simulink model "sampleModel2199"  (R2022a)
settings: Solver=FixedStepAuto  StartTime=0.0  StopTime=10.0  RelTol=1e-3
undefined symbols (not defined in the file): DiscIntNeverNeededParam, Newton, Raphson
libraries: simulink x64, slpidlib x16
(part 1 of 3)
settings Model: SimulationMode=software-in-the-loop (sil)  Creator=lenovo  LastModifiedBy=TSMC
settings DataIOCC: InspectSignalLogs=on  SignalLoggingName=logsOut
settings OptimizationCC: DefaultParameterBehavior=Inlined  EnhancedBackFolding=on  PassReuseOutputArgsAs=Individual arguments  ZeroExternalMemoryAtStartup=off  ZeroInternalMemoryAtStartup=off  OptimizeBlockOrder=speed  DifferentSizesBufferReuse=on  OptimizationCustomize=off  EfficientTunableParamExpr=on
settings DebuggingCC: ParameterTunabilityLossMsg=error  UnconnectedInputMsg=warning  UnconnectedOutputMsg=warning  UnconnectedLineMsg=warning
settings ModelReferenceCC: UpdateModelReferenceTargets=Force
settings SFSimCC: MATLABDynamicMemAlloc=off
settings RTWCC: SystemTargetFile=ert.tlc  TemplateMakefile=ert_default_tmf  GenerateReport=on  IncludeHyperlinkInReport=on  GenerateTraceInfo=on  DLArmComputeVersion=19.05
settings CodeAppCC: ForceParamTrailComments=on  IgnoreCustomStorageClasses=off  OperatorAnnotations=on  SimulinkDataObjDesc=on  SFDataObjDesc=on  InsertBlockDesc=on
settings ERTTargetCC: TargetLangStandard=C99 (ISO)  GenerateSampleERTMain=on  SupportContinuousTime=on  InlinedParameterPlacement=NonHierarchical  ERTCustomFileTemplate=example_file_process.tlc

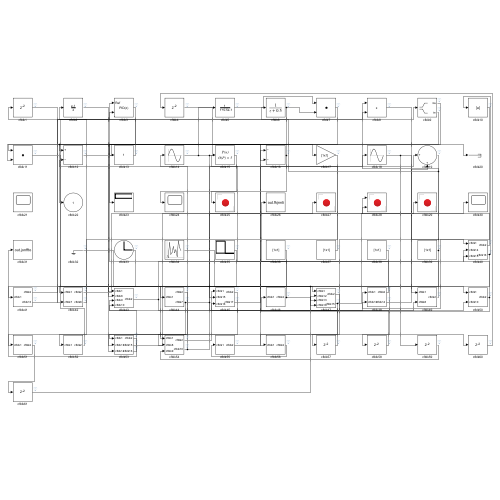
[thumbnail: Simulink's stored preview of the top-level diagram]
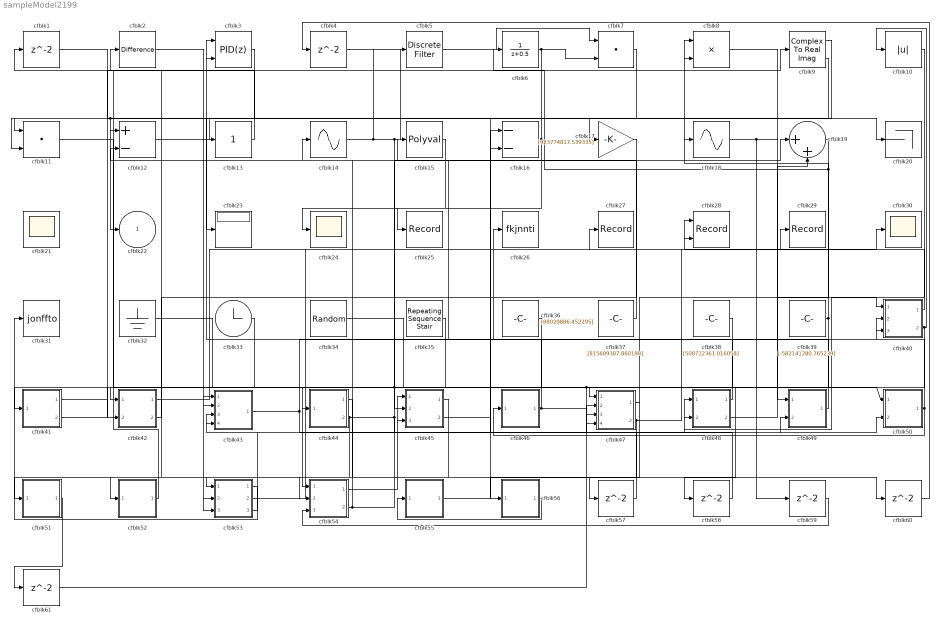
== system sampleModel2199 ==
  cfblk{1,4,57..61} (7 alike) : Delay  SampleTime=1
  cfblk10 : Abs  SaturateOnIntegerOverflow=off
  cfblk11 : DotProduct  OutDataTypeStr=Inherit: Inherit via internal rule
  cfblk12 : Sum  Inputs=+-
  cfblk13 : simulink/Math Operations/Slider Gain  gain=1  low=0  high=2
  cfblk14 : Sin  TimeSource=Use external signal  SampleTime=0
  cfblk15 : Polyval  Coefs=[ +2.081618890e-019, -1.441693666e-014, +4.719686976e-010, -8.536869453e-006, +1.621573104e-001, -8.087801117e+001 ]
  cfblk16 : Sum  Inputs=--
  cfblk17 : Gain  Gain=[923774817.539335]
  cfblk18 : Sin  TimeSource=Use external signal  SampleTime=0
  cfblk19 : Sum  Inputs=|++
  cfblk2 : simulink/Discrete/Difference  ICPrevInput=0.0  OutMin=[]  OutMax=[]  OutDataTypeStr=Inherit: Inherit via back propagation  OutDataType=fixdt(1, 16)  OutScaling=2^-10  DoSatur=off
  cfblk20 : Terminator
  cfblk21 : Scope
      settings: Floating=on
  cfblk23 : Display
  cfblk24 : Scope
  cfblk25 : Record  FileSettingsInternal="{\"entries\":[{\"content\":{\"excelSettings\":{\"content\":{},\"type\":\"Streamout.ExcelSettings\"}},\"type\":\"Streamout.FileSettingStorage\",\"uuid\":\"e2bdf832-fa04-45a0-9737-202340bf4c1e\"}],\"packageUris\":[\"http://schema.mathworks.com/mf0/streamout_blocks/R2020a\"],\"version\":\"1.0\"}"  SignalsInternal="{\"entries\":[{\"content\":{\"signals\":[]},\"type\":\"RecordBlkView.InputSignals\",\"uuid\":\"caab4e54-0413-4384-8605-d26ba1fc89d5\"}],\"packageUris\":[\"http://schema.mathworks.com/mf0/streamout_blocks/R2020a\"],\"version\":\"1.0\"}"  VisualizationBindings="{\"sparklinesplugin\":{\"info\":[{\"bindingParametersList\":[],\"subplotID\":1}]}}"
  cfblk26 : ToWorkspace  VariableName=fkjnnti  SaveFormat=Timeseries  SampleTime=-1
  cfblk27 : Record  FileSettingsInternal="{\"entries\":[{\"content\":{\"excelSettings\":{\"content\":{},\"type\":\"Streamout.ExcelSettings\"}},\"type\":\"Streamout.FileSettingStorage\",\"uuid\":\"b3a37654-cf2f-4752-9820-15f634001c55\"}],\"packageUris\":[\"http://schema.mathworks.com/mf0/streamout_blocks/R2020a\"],\"version\":\"1.0\"}"  SignalsInternal="{\"entries\":[{\"content\":{\"signals\":[]},\"type\":\"RecordBlkView.InputSignals\",\"uuid\":\"67388c61-a990-4278-b841-d462b1e08af4\"}],\"packageUris\":[\"http://schema.mathworks.com/mf0/streamout_blocks/R2020a\"],\"version\":\"1.0\"}"  VisualizationBindings="{\"sparklinesplugin\":{\"info\":[{\"bindingParametersList\":[],\"subplotID\":1}]}}"
  cfblk28 : Record  FileSettingsInternal="{\"entries\":[{\"content\":{\"excelSettings\":{\"content\":{},\"type\":\"Streamout.ExcelSettings\"}},\"type\":\"Streamout.FileSettingStorage\",\"uuid\":\"9d0e44ae-21f0-49fd-83ab-d770f6f5ba27\"}],\"packageUris\":[\"http://schema.mathworks.com/mf0/streamout_blocks/R2020a\"],\"version\":\"1.0\"}"  Layout=[1 1]  SignalsInternal="{\"entries\":[{\"content\":{\"signals\":[]},\"type\":\"RecordBlkView.InputSignals\",\"uuid\":\"6b70960c-b6c1-44c9-85c3-124069d1ad3e\"}],\"packageUris\":[\"http://schema.mathworks.com/mf0/streamout_blocks/R2020a\"],\"version\":\"1.0\"}"  VisualizationBindings="{\"xyplotplugin\":{\"info\":[{\"series\":[],\"subplotID\":1}]}}"  CompatibilityTag=XY  st=-1
  cfblk29 : Record  FileSettingsInternal="{\"entries\":[{\"content\":{\"excelSettings\":{\"content\":{},\"type\":\"Streamout.ExcelSettings\"}},\"type\":\"Streamout.FileSettingStorage\",\"uuid\":\"98bdaffd-6e83-499c-ad62-c427105a1288\"}],\"packageUris\":[\"http://schema.mathworks.com/mf0/streamout_blocks/R2020a\"],\"version\":\"1.0\"}"  SignalsInternal="{\"entries\":[{\"content\":{\"signals\":[]},\"type\":\"RecordBlkView.InputSignals\",\"uuid\":\"ff5ee5ea-edd2-48fc-8483-bfde92b337d5\"}],\"packageUris\":[\"http://schema.mathworks.com/mf0/streamout_blocks/R2020a\"],\"version\":\"1.0\"}"  VisualizationBindings="{\"sparklinesplugin\":{\"info\":[{\"bindingParametersList\":[],\"subplotID\":1}]}}"
  cfblk3 : slpidlib/PID Controller (2DOF)  Controller=PID  Form=Parallel  TimeDomain=Discrete-time  UseExternalTs=off  SampleTime=1  IntegratorMethod=Forward Euler  FilterMethod=Forward Euler  ControllerParametersSource=internal  P=1  I=1  UseKiTs=off  D=0  N=100  UseFilter=on  b=1  c=1  TunerSelectOption=Transfer Function Based (PID Tuner App)  InitialConditionSource=internal  InitialConditionForIntegrator=0  InitialConditionForFilter=0  DifferentiatorICPrevScaledInput=0  ExternalReset=none  TrackingMode=off  Kt=1  LimitOutput=off  SatLimitsSource=internal  UpperSaturationLimit=inf  LowerSaturationLimit=-inf  LinearizeAsGain=off  AntiWindupMode=none  Kb=1  POutMin=[]  POutMax=[]  IOutMin=[]  IOutMax=[]  DOutMin=[]  DOutMax=[]  NOutMin=[]  NOutMax=[]  bOutMin=[]  bOutMax=[]  cOutMin=[]  cOutMax=[]  SumOutMin=[]  SumOutMax=[]  SaturationOutMin=[]  SaturationOutMax=[]  PParamMin=[]  PParamMax=[]  IParamMin=[]  IParamMax=[]  DParamMin=[]  DParamMax=[]  NParamMin=[]  NParamMax=[]  bParamMin=[]  bParamMax=[]  cParamMin=[]  cParamMax=[]  KbParamMin=[]  KbParamMax=[]  KtParamMin=[]  KtParamMax=[]  KbOutMin=[]  KbOutMax=[]  KtOutMin=[]  KtOutMax=[]  IntegratorOutMin=[]  IntegratorOutMax=[]  FilterOutMin=[]  FilterOutMax=[]  SumI1OutMin=[]  SumI1OutMax=[]  SumI2OutMin=[]  SumI2OutMax=[]  SumI3OutMin=[]  SumI3OutMax=[]  SumI4OutMin=[]  SumI4OutMax=[]  SumDOutMin=[]  SumDOutMax=[]  Sum1OutMin=[]  Sum1OutMax=[]  Sum2OutMin=[]  Sum2OutMax=[]  Sum3OutMin=[]  Sum3OutMax=[]  DifferentiatorOutMin=[]  DifferentiatorOutMax=[]  FilterDiffOutCoefMin=[]  FilterDiffOutCoefMax=[]  ReciprocalOutMin=[]  ReciprocalOutMax=[]  SumDenOutMin=[]  SumDenOutMax=[]  SumNumOutMin=[]  SumNumOutMax=[]  DivideOutMin=[]  DivideOutMax=[]  UdiffTsProdOutMin=[]  UdiffTsProdOutMax=[]  NTsProdOutMin=[]  NTsProdOutMax=[]  UintegralTsProdOutMin=[]  UintegralTsProdOutMax=[]  UngainTsProdOutMin=[]  UngainTsProdOutMax=[]  IntegratorContinuousStateAttributes=''  IntegratorStateMustResolveToSignalObject=off  IntegratorRTWStateStorageClass=Auto  FilterContinuousStateAttributes=''  FilterStateMustResolveToSignalObject=off  FilterRTWStateStorageClass=Auto  ParallelPVariant=InternalParameters  IdealPVariant=Disabled  IVariant=InternalParameters  DVariant=InternalParameters  bVariant=InternalParameters  cVariant=InternalParameters  IntegratorVariant=Discrete  SatVariant=Disabled  AWVariant=Passthrough  PCopyVariant=Disabled  TRVariant=Disabled  FdbkBlocksVariant=Forward  IdealPFdbkVariant=Disabled  SatFdbkVariant=Disabled  DerivativeFilterVariant=ForwardEulerFilter  NVariant=InternalParameters  NCopyVariant=Disabled  FilterICVariant=InternalICsFilter  IntegratorICVariant=InternalICs  ExternalResetVariant=Disabled  TRSumVariant=Passthrough  SumFdbkVariant=Disabled  SumVariant=Sum_PID  TsampFilterVariant=InternalTs  TsampNgainVariant=Passthrough  TsampIntegralVariant=Passthrough  ExternalSaturationOutDataTypeStr=Inherit: Same as second input
      settings: SourceProductBaseCode=SL
  cfblk30 : Scope
  cfblk31 : ToWorkspace  VariableName=jonffto  SaveFormat=Timeseries  SampleTime=-1
  cfblk32 : Ground
  cfblk33 : Clock
  cfblk34 : UniformRandomNumber  Minimum=[-4540593031.806434]  Maximum=[3282610122.019338]  Seed=[18241639.000000]  SampleTime=0.1
  cfblk35 : simulink/Sources/Repeating Sequence Stair  OutValues=[891316863.634879, -8817081.517770]  tsamp=-1  OutMin=[]  OutMax=[]  OutDataTypeStr=double  OutputDataTypeScalingMode=double  OutDataType=fixdt(0,8)  ConRadixGroup=Best Precision: Vector-wise  OutScaling=2^-12
  cfblk36 : Constant  Value=[88029886.452295]  SampleTime=1
  cfblk37 : Constant  Value=[815609387.860188]  SampleTime=1
  cfblk38 : Constant  Value=[508712361.016058]  SampleTime=1
  cfblk39 : Constant  Value=[-582141280.765239]  SampleTime=1
  cfblk40 : Subsystem
  cfblk41 : Subsystem
  cfblk42 : Subsystem
  cfblk43 : Subsystem
  cfblk44 : Subsystem
  cfblk45 : Subsystem
  cfblk46 : Subsystem
  cfblk47 : Subsystem
  cfblk48 : Subsystem
  cfblk49 : Subsystem
  cfblk5 : DiscreteFilter  SampleTime=1
  cfblk50 : Subsystem
  cfblk51 : Subsystem
  cfblk52 : Subsystem
  cfblk53 : Subsystem
  cfblk54 : Subsystem
  cfblk55 : Subsystem
  cfblk56 : Subsystem
  cfblk6 : DiscreteTransferFcn  SampleTime=1
  cfblk7 : DotProduct  OutDataTypeStr=Inherit: Inherit via internal rule
  cfblk8 : Product
  cfblk9 : ComplexToRealImag
  cfblk22 : Outport
  wires:
  cfblk12/1 -> cfblk20/1
  cfblk52/1(cfblk2) -> cfblk8/1
  cfblk39/1 -> cfblk53/3(cfblk14), cfblk47/4(cfblk14), cfblk8/2, cfblk6/1
  cfblk15/1 -> cfblk25/1
  cfblk54/1(cfblk2) -> cfblk45/1(cfblk1)
  cfblk53/1(cfblk2) -> cfblk31/1
  cfblk35/1 -> cfblk41/1(cfblk1)
  cfblk16/1 -> cfblk24/1, cfblk11/1
  cfblk53/2(cfblk15) -> cfblk28/1
  cfblk36/1 -> cfblk42/1(cfblk1)
  cfblk42/1(cfblk2) -> cfblk29/1
  cfblk48/1(cfblk2) -> cfblk3/1
  cfblk11/1 -> cfblk54/1(cfblk1)
  cfblk38/1 -> cfblk44/1(cfblk1)
  cfblk56/1(cfblk2) -> cfblk55/1(cfblk1)
  cfblk3/1 -> cfblk23/1
  cfblk42/2(cfblk8) -> cfblk2/1
  cfblk14/1 -> cfblk17/1, cfblk47/3(cfblk13), cfblk5/1
  cfblk17/1 -> cfblk52/1(cfblk1)
  cfblk1/1 -> cfblk16/2
  cfblk2/1 -> cfblk43/1(cfblk1)
  cfblk6/1 -> cfblk22/1, cfblk11/2, cfblk7/2
  cfblk41/1(cfblk2) -> cfblk3/2
  cfblk10/1 -> cfblk48/1(cfblk1)
  cfblk46/1(cfblk2) -> cfblk26/1, cfblk48/2(cfblk13)
  cfblk7/1 -> cfblk43/2(cfblk8)
  cfblk8/1 -> cfblk49/1(cfblk1)
  cfblk45/1(cfblk2) -> cfblk53/1(cfblk1)
  cfblk33/1 -> cfblk42/2(cfblk7)
  cfblk41/2(cfblk13) -> cfblk9/1
  cfblk37/1 -> cfblk14/1
  cfblk9/1 -> cfblk13/1
  cfblk50/1(cfblk2) -> cfblk46/1(cfblk1), cfblk40/3(cfblk15)
  cfblk43/1(cfblk2) -> cfblk49/2(cfblk8), cfblk40/2(cfblk14)
  cfblk49/1(cfblk2) -> cfblk15/1
  cfblk4/1 -> cfblk56/1(cfblk1)
  cfblk40/1(cfblk2) -> cfblk28/2
  cfblk44/1(cfblk2) -> cfblk53/2(cfblk13)
  cfblk9/2 -> cfblk12/1
  cfblk53/3(cfblk16) -> cfblk43/3(cfblk9)
  cfblk13/1 -> cfblk1/1
  cfblk40/2(cfblk16) -> cfblk10/1, cfblk58/1
  cfblk54/2(cfblk10) -> cfblk19/1, cfblk12/2
  cfblk48/2(cfblk14) -> cfblk19/2
  cfblk34/1 -> cfblk47/1(cfblk1)
  cfblk44/2(cfblk7) -> cfblk50/1(cfblk1), cfblk27/1, cfblk50/2(cfblk10), cfblk54/2(cfblk8)
  cfblk18/1 -> cfblk40/1(cfblk1), cfblk59/1
  cfblk45/2(cfblk17) -> cfblk18/1
  cfblk5/1 -> cfblk7/1
  cfblk32/1 -> cfblk45/2(cfblk15)
  cfblk47/1(cfblk2) -> cfblk43/4(cfblk10)
  cfblk47/2(cfblk15) -> cfblk30/1, cfblk51/1(cfblk1)
  cfblk19/1 -> cfblk57/1
  cfblk57/1 -> cfblk16/1
  cfblk58/1 -> cfblk45/3(cfblk16)
  cfblk59/1 -> cfblk54/3(cfblk9)
  cfblk55/1(cfblk2) -> cfblk60/1
  cfblk60/1 -> cfblk4/1
  cfblk51/1(cfblk2) -> cfblk61/1
  cfblk61/1 -> cfblk47/2(cfblk12)

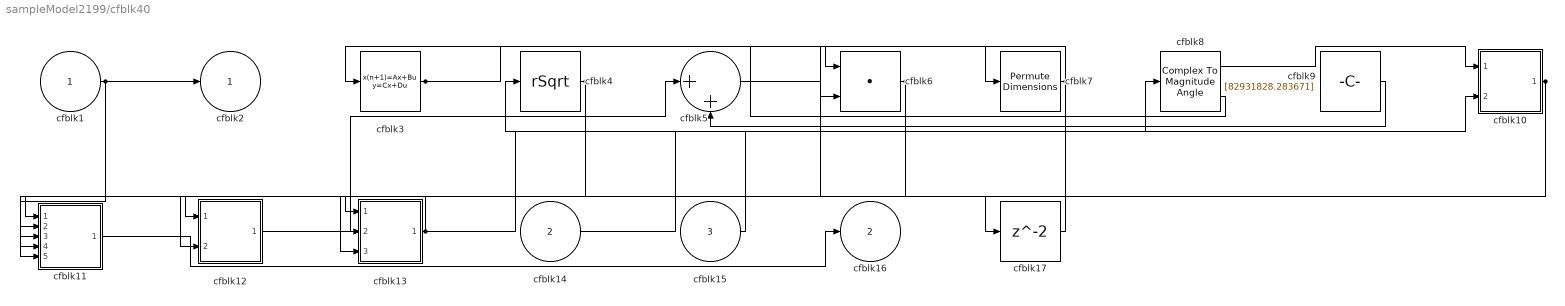
== system sampleModel2199/cfblk40 ==
  cfblk1 : Inport
  cfblk14 : Inport  Port=2
  cfblk15 : Inport  Port=3
  cfblk10 : Subsystem
  cfblk11 : Subsystem
  cfblk12 : Subsystem
  cfblk13 : Subsystem
  cfblk17 : Delay  SampleTime=1
  cfblk3 : DiscreteStateSpace
  cfblk4 : Sqrt  Operator=rSqrt  AlgorithmType=Newton-Raphson
  cfblk5 : Sum  Inputs=|++
  cfblk6 : DotProduct  OutDataTypeStr=Inherit: Inherit via internal rule
  cfblk7 : PermuteDimensions
  cfblk8 : ComplexToMagnitudeAngle
  cfblk9 : Constant  Value=[82931828.283671]  SampleTime=1
  cfblk2 : Outport
  cfblk16 : Outport  Port=2
  wires:
  cfblk10/1(cfblk2) -> cfblk11/1(cfblk1), cfblk11/5(cfblk12)
  cfblk8/1 -> cfblk10/1(cfblk1)
  cfblk1/1 -> cfblk2/1, cfblk11/4(cfblk11)
  cfblk12/1(cfblk2) -> cfblk5/1
  cfblk9/1 -> cfblk5/2
  cfblk4/1 -> cfblk13/1(cfblk1), cfblk13/2(cfblk11)
  cfblk8/2 -> cfblk3/1
  cfblk11/1(cfblk2) -> cfblk16/1
  cfblk15/1 -> cfblk4/1
  cfblk14/1 -> cfblk8/1
  cfblk3/1 -> cfblk7/1, cfblk6/2
  cfblk7/1 -> cfblk12/2(cfblk11), cfblk6/1
  cfblk13/1(cfblk2) -> cfblk10/2(cfblk15), cfblk11/3(cfblk10)
  cfblk6/1 -> cfblk11/2(cfblk9), cfblk13/3(cfblk12)
  cfblk5/1 -> cfblk17/1
  cfblk17/1 -> cfblk12/1(cfblk1)

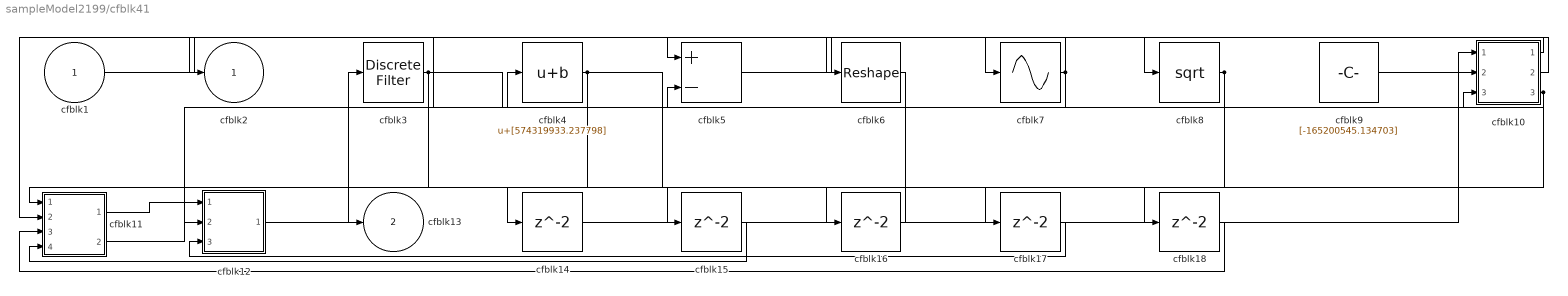
== system sampleModel2199/cfblk41 ==
  cfblk1 : Inport
  cfblk10 : Subsystem
  cfblk11 : Subsystem
  cfblk12 : Subsystem
  cfblk{14..18} (5 alike) : Delay  SampleTime=1
  cfblk3 : DiscreteFilter  SampleTime=1
  cfblk4 : Bias  Bias=[574319933.237798]  SaturateOnIntegerOverflow=off
  cfblk5 : Sum  Inputs=+-
  cfblk6 : Reshape
  cfblk7 : Sin  TimeSource=Use external signal  SampleTime=0
  cfblk8 : Sqrt
  cfblk9 : Constant  Value=[-165200545.134703]  SampleTime=1
  cfblk2 : Outport
  cfblk13 : Outport  Port=2
  wires:
  cfblk8/1 -> cfblk16/1, cfblk17/1
  cfblk5/1 -> cfblk8/1
  cfblk12/1(cfblk2) -> cfblk3/1
  cfblk7/1 -> cfblk11/2(cfblk12), cfblk5/1
  cfblk1/1 -> cfblk7/1
  cfblk9/1 -> cfblk10/2(cfblk11)
  cfblk10/1(cfblk2) -> cfblk2/1
  cfblk10/2(cfblk13) -> cfblk6/1
  cfblk4/1 -> cfblk12/2(cfblk11), cfblk18/1
  cfblk10/3(cfblk14) -> cfblk5/2, cfblk15/1
  cfblk11/1(cfblk2) -> cfblk12/1(cfblk1)
  cfblk11/2(cfblk15) -> cfblk4/1
  cfblk3/1 -> cfblk10/3(cfblk12), cfblk13/1
  cfblk6/1 -> cfblk14/1
  cfblk14/1 -> cfblk10/1(cfblk1)
  cfblk15/1 -> cfblk11/4(cfblk14)
  cfblk16/1 -> cfblk11/1(cfblk1)
  cfblk17/1 -> cfblk12/3(cfblk12)
  cfblk18/1 -> cfblk11/3(cfblk13)

== system sampleModel2199/cfblk42 ==
  cfblk1 : Inport
  cfblk7 : Inport  Port=2
  cfblk3 : simulink/Discrete/Transfer Fcn Lead or Lag  PoleZ=0.95  ZeroZ=0.75  ICPrevOutput=0.0  ICPrevInput=0.0  DoSatur=off
      settings: SourceProductBaseCode=SL
  cfblk4 : simulink/Discrete/Difference  ICPrevInput=0.0  OutMin=[]  OutMax=[]  OutDataTypeStr=Inherit: Inherit via back propagation  OutDataType=fixdt(1, 16)  OutScaling=2^-10  DoSatur=off
  cfblk5 : MinMax  Function=max
  cfblk6 : Reshape
  cfblk2 : Outport
  cfblk8 : Outport  Port=2
  wires:
  cfblk5/1 -> cfblk8/1
  cfblk1/1 -> cfblk6/1
  cfblk6/1 -> cfblk3/1
  cfblk3/1 -> cfblk5/1
  cfblk7/1 -> cfblk4/1
  cfblk4/1 -> cfblk2/1

== system sampleModel2199/cfblk43 ==
  cfblk1 : Inport
  cfblk8 : Inport  Port=2
  cfblk9 : Inport  Port=3
  cfblk10 : Inport  Port=4
  cfblk11 : Delay  SampleTime=1
  cfblk3 : simulink/Discrete/Difference  ICPrevInput=0.0  OutMin=[]  OutMax=[]  OutDataTypeStr=Inherit: Inherit via back propagation  OutDataType=fixdt(1, 16)  OutScaling=2^-10  DoSatur=off
  cfblk4 : simulink/Discrete/Transfer Fcn Lead or Lag  PoleZ=0.95  ZeroZ=0.75  ICPrevOutput=0.0  ICPrevInput=0.0  DoSatur=off
      settings: SourceProductBaseCode=SL
  cfblk5 : Sqrt  Operator=rSqrt  AlgorithmType=Newton-Raphson
  cfblk6 : Squeeze
  cfblk7 : Subsystem
  cfblk2 : Outport
  wires:
  cfblk10/1 -> cfblk5/1
  cfblk8/1 -> cfblk6/1, cfblk7/4(cfblk10)
  cfblk3/1 -> cfblk4/1, cfblk7/5(cfblk11)
  cfblk9/1 -> cfblk7/1(cfblk1)
  cfblk1/1 -> cfblk2/1
  cfblk5/1 -> cfblk7/2(cfblk8)
  cfblk6/1 -> cfblk7/3(cfblk9)
  cfblk4/1 -> cfblk11/1
  cfblk11/1 -> cfblk3/1

== system sampleModel2199/cfblk44 ==
  cfblk1 : Inport
  cfblk10 : Delay  SampleTime=1
  cfblk3 : Reshape
  cfblk4 : DotProduct  OutDataTypeStr=Inherit: Inherit via internal rule
  cfblk5 : Subsystem
  cfblk6 : Subsystem
  cfblk8 : Delay  SampleTime=1
  cfblk9 : Delay  SampleTime=1
  cfblk2 : Outport
  cfblk7 : Outport  Port=2
  wires:
  cfblk6/1(cfblk2) -> cfblk7/1
  cfblk1/1 -> cfblk4/1, cfblk6/5(cfblk16)
  cfblk5/1(cfblk2) -> cfblk6/1(cfblk1)
  cfblk3/1 -> cfblk6/3(cfblk14), cfblk10/1
  cfblk6/2(cfblk17) -> cfblk8/1, cfblk9/1
  cfblk4/1 -> cfblk2/1, cfblk5/2(cfblk7)
  cfblk5/2(cfblk9) -> cfblk6/2(cfblk13)
  cfblk5/3(cfblk10) -> cfblk3/1, cfblk6/4(cfblk15)
  cfblk8/1 -> cfblk5/1(cfblk1)
  cfblk9/1 -> cfblk5/3(cfblk8)
  cfblk10/1 -> cfblk4/2

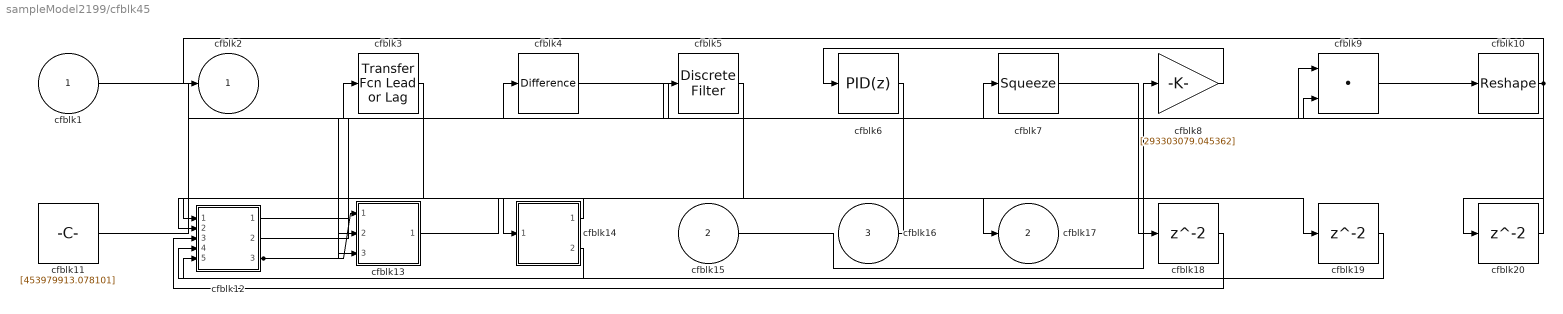
== system sampleModel2199/cfblk45 ==
  cfblk1 : Inport
  cfblk15 : Inport  Port=2
  cfblk16 : Inport  Port=3
  cfblk10 : Reshape
  cfblk11 : Constant  Value=[453979913.078101]  SampleTime=1
  cfblk12 : Subsystem
  cfblk13 : Subsystem
  cfblk14 : Subsystem
  cfblk18 : Delay  SampleTime=1
  cfblk19 : Delay  SampleTime=1
  cfblk20 : Delay  SampleTime=1
  cfblk3 : simulink/Discrete/Transfer Fcn Lead or Lag  PoleZ=0.95  ZeroZ=0.75  ICPrevOutput=0.0  ICPrevInput=0.0  DoSatur=off
      settings: SourceProductBaseCode=SL
  cfblk4 : simulink/Discrete/Difference  ICPrevInput=0.0  OutMin=[]  OutMax=[]  OutDataTypeStr=Inherit: Inherit via back propagation  OutDataType=fixdt(1, 16)  OutScaling=2^-10  DoSatur=off
  cfblk5 : DiscreteFilter  SampleTime=1
  cfblk6 : slpidlib/PID Controller  Controller=PID  Form=Parallel  TimeDomain=Discrete-time  UseExternalTs=off  SampleTime=1  IntegratorMethod=Forward Euler  FilterMethod=Forward Euler  ControllerParametersSource=internal  P=1  I=1  UseKiTs=off  D=0  N=100  UseFilter=on  TunerSelectOption=Transfer Function Based (PID Tuner App)  InitialConditionSource=internal  InitialConditionForIntegrator=0  InitialConditionForFilter=0  DifferentiatorICPrevScaledInput=0  ExternalReset=none  TrackingMode=off  Kt=1  LimitOutput=off  SatLimitsSource=internal  UpperSaturationLimit=inf  LowerSaturationLimit=-inf  LinearizeAsGain=off  AntiWindupMode=none  Kb=1  POutMin=[]  POutMax=[]  IOutMin=[]  IOutMax=[]  DOutMin=[]  DOutMax=[]  NOutMin=[]  NOutMax=[]  SumOutMin=[]  SumOutMax=[]  SaturationOutMin=[]  SaturationOutMax=[]  PParamMin=[]  PParamMax=[]  IParamMin=[]  IParamMax=[]  DParamMin=[]  DParamMax=[]  NParamMin=[]  NParamMax=[]  KbParamMin=[]  KbParamMax=[]  KtParamMin=[]  KtParamMax=[]  KbOutMin=[]  KbOutMax=[]  KtOutMin=[]  KtOutMax=[]  IntegratorOutMin=[]  IntegratorOutMax=[]  FilterOutMin=[]  FilterOutMax=[]  SumI1OutMin=[]  SumI1OutMax=[]  SumI2OutMin=[]  SumI2OutMax=[]  SumI3OutMin=[]  SumI3OutMax=[]  SumI4OutMin=[]  SumI4OutMax=[]  SumDOutMin=[]  SumDOutMax=[]  DifferentiatorOutMin=[]  DifferentiatorOutMax=[]  FilterDiffOutCoefMin=[]  FilterDiffOutCoefMax=[]  ReciprocalOutMin=[]  ReciprocalOutMax=[]  SumDenOutMin=[]  SumDenOutMax=[]  SumNumOutMin=[]  SumNumOutMax=[]  DivideOutMin=[]  DivideOutMax=[]  UdiffTsProdOutMin=[]  UdiffTsProdOutMax=[]  NTsProdOutMin=[]  NTsProdOutMax=[]  UintegralTsProdOutMin=[]  UintegralTsProdOutMax=[]  UngainTsProdOutMin=[]  UngainTsProdOutMax=[]  IntegratorContinuousStateAttributes=''  IntegratorStateMustResolveToSignalObject=off  IntegratorRTWStateStorageClass=Auto  FilterContinuousStateAttributes=''  FilterStateMustResolveToSignalObject=off  FilterRTWStateStorageClass=Auto  ParallelPVariant=InternalParameters  IdealPVariant=Disabled  IVariant=InternalParameters  DVariant=InternalParameters  IntegratorVariant=Discrete  SatVariant=Disabled  AWVariant=Passthrough  PCopyVariant=Disabled  TRVariant=Disabled  FdbkBlocksVariant=Forward  IdealPFdbkVariant=Disabled  SatFdbkVariant=Disabled  DerivativeFilterVariant=ForwardEulerFilter  NVariant=InternalParameters  NCopyVariant=Disabled  FilterICVariant=InternalICsFilter  IntegratorICVariant=InternalICs  ExternalResetVariant=Disabled  TRSumVariant=Passthrough  SumFdbkVariant=Disabled  SumVariant=Sum_PID  TsampFilterVariant=InternalTs  TsampNgainVariant=Passthrough  TsampIntegralVariant=Passthrough  ExternalSaturationOutDataTypeStr=Inherit: Same as second input  aMode=0
  cfblk7 : Squeeze
  cfblk8 : Gain  Gain=[293303079.045362]
  cfblk9 : DotProduct  OutDataTypeStr=Inherit: Inherit via internal rule
  cfblk2 : Outport
  cfblk17 : Outport  Port=2
  wires:
  cfblk8/1 -> cfblk6/1
  cfblk4/1 -> cfblk7/1
  cfblk9/1 -> cfblk10/1
  cfblk12/1(cfblk2) -> cfblk17/1
  cfblk11/1 -> cfblk3/1
  cfblk15/1 -> cfblk8/1
  cfblk1/1 -> cfblk14/1(cfblk1)
  cfblk16/1 -> cfblk5/1
  cfblk10/1 -> cfblk2/1, cfblk20/1
  cfblk12/2(cfblk13) -> cfblk4/1
  cfblk14/1(cfblk2) -> cfblk12/1(cfblk1)
  cfblk12/3(cfblk14) -> cfblk13/1(cfblk1), cfblk9/2
  cfblk6/1 -> cfblk13/2(cfblk10)
  cfblk5/1 -> cfblk12/2(cfblk9)
  cfblk3/1 -> cfblk13/3(cfblk11)
  cfblk14/2(cfblk10) -> cfblk12/5(cfblk12)
  cfblk7/1 -> cfblk18/1
  cfblk18/1 -> cfblk12/3(cfblk10)
  cfblk13/1(cfblk2) -> cfblk19/1
  cfblk19/1 -> cfblk12/4(cfblk11)
  cfblk20/1 -> cfblk9/1

== system sampleModel2199/cfblk46 ==
  cfblk1 : Inport
  cfblk{8..12} (5 alike) : Delay  SampleTime=1
  cfblk3 : simulink/Discrete/Tapped Delay  vinit=0.0  samptime=-1  NumDelays=1  DelayOrder=Oldest  includeCurrent=off
  cfblk4 : Subsystem
  cfblk5 : Subsystem
  cfblk6 : Subsystem
  cfblk7 : Subsystem
  cfblk2 : Outport
  wires:
  cfblk1/1 -> cfblk6/2(cfblk7), cfblk5/2(cfblk10), cfblk7/4(cfblk13), cfblk7/6(cfblk15)
  cfblk6/1(cfblk2) -> cfblk3/1, cfblk5/1(cfblk1), cfblk4/4(cfblk13)
  cfblk7/1(cfblk2) -> cfblk4/1(cfblk1)
  cfblk5/2(cfblk11) -> cfblk4/2(cfblk11), cfblk7/5(cfblk14)
  cfblk3/1 -> cfblk7/1(cfblk1)
  cfblk4/2(cfblk14) -> cfblk9/1, cfblk10/1, cfblk11/1
  cfblk7/2(cfblk17) -> cfblk2/1, cfblk4/3(cfblk12)
  cfblk4/1(cfblk2) -> cfblk8/1
  cfblk8/1 -> cfblk6/1(cfblk1)
  cfblk9/1 -> cfblk7/2(cfblk11)
  cfblk10/1 -> cfblk7/3(cfblk12)
  cfblk11/1 -> cfblk7/7(cfblk16)
  cfblk5/1(cfblk2) -> cfblk12/1
  cfblk12/1 -> cfblk6/3(cfblk8)

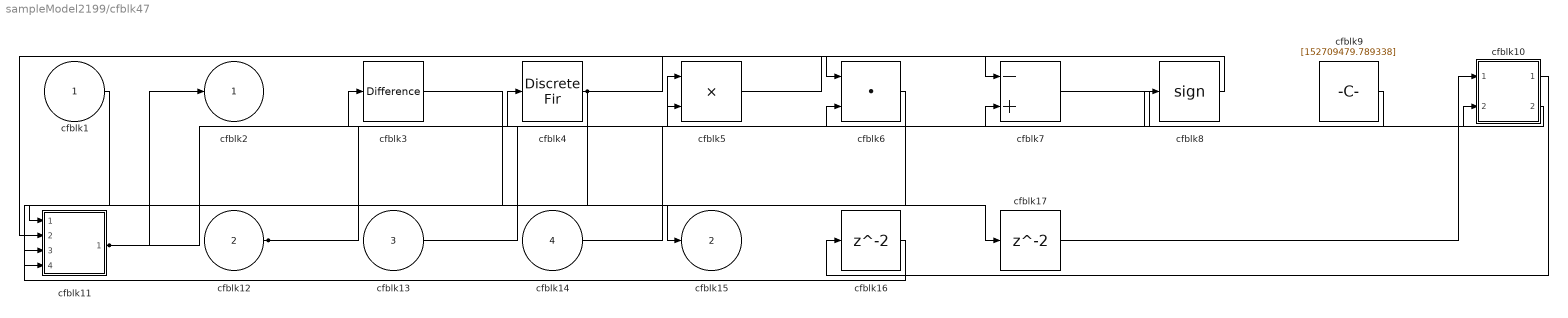
== system sampleModel2199/cfblk47 ==
  cfblk1 : Inport
  cfblk12 : Inport  Port=2
  cfblk13 : Inport  Port=3
  cfblk14 : Inport  Port=4
  cfblk10 : Subsystem
  cfblk11 : Subsystem
  cfblk16 : Delay  SampleTime=1
  cfblk17 : Delay  SampleTime=1
  cfblk3 : simulink/Discrete/Difference  ICPrevInput=0.0  OutMin=[]  OutMax=[]  OutDataTypeStr=Inherit: Inherit via back propagation  OutDataType=fixdt(1, 16)  OutScaling=2^-10  DoSatur=off
  cfblk4 : DiscreteFir  SampleTime=1
  cfblk5 : Product
  cfblk6 : DotProduct  OutDataTypeStr=Inherit: Inherit via internal rule
  cfblk7 : Sum  Inputs=-+
  cfblk8 : Signum
  cfblk9 : Constant  Value=[152709479.789338]  SampleTime=1
  cfblk2 : Outport
  cfblk15 : Outport  Port=2
  wires:
  cfblk11/1(cfblk2) -> cfblk2/1, cfblk7/2
  cfblk13/1 -> cfblk5/1
  cfblk1/1 -> cfblk11/1(cfblk1)
  cfblk12/1 -> cfblk4/1, cfblk8/1
  cfblk6/1 -> cfblk15/1
  cfblk8/1 -> cfblk11/2(cfblk13)
  cfblk4/1 -> cfblk6/1, cfblk11/4(cfblk15)
  cfblk5/1 -> cfblk7/1
  cfblk9/1 -> cfblk5/2
  cfblk14/1 -> cfblk6/2
  cfblk10/2(cfblk9) -> cfblk3/1
  cfblk7/1 -> cfblk10/2(cfblk8)
  cfblk10/1(cfblk2) -> cfblk16/1
  cfblk16/1 -> cfblk11/3(cfblk14)
  cfblk3/1 -> cfblk17/1
  cfblk17/1 -> cfblk10/1(cfblk1)

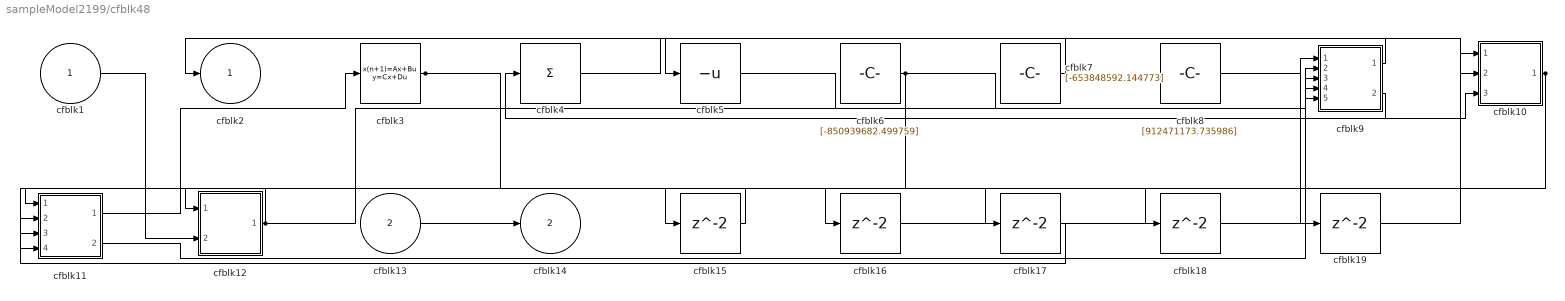
== system sampleModel2199/cfblk48 ==
  cfblk1 : Inport
  cfblk13 : Inport  Port=2
  cfblk10 : Subsystem
  cfblk11 : Subsystem
  cfblk12 : Subsystem
  cfblk{15..19} (5 alike) : Delay  SampleTime=1
  cfblk3 : DiscreteStateSpace
  cfblk4 : Sum  Inputs=+
  cfblk5 : UnaryMinus
  cfblk6 : Constant  Value=[-850939682.499759]  SampleTime=1
  cfblk7 : Constant  Value=[-653848592.144773]  SampleTime=1
  cfblk8 : Constant  Value=[912471173.735986]  SampleTime=1
  cfblk9 : Subsystem
  cfblk2 : Outport
  cfblk14 : Outport  Port=2
  wires:
  cfblk9/1(cfblk2) -> cfblk2/1
  cfblk10/1(cfblk2) -> cfblk11/1(cfblk1), cfblk15/1
  cfblk13/1 -> cfblk14/1
  cfblk3/1 -> cfblk16/1, cfblk17/1, cfblk18/1
  cfblk12/1(cfblk2) -> cfblk9/2(cfblk13), cfblk11/2(cfblk13)
  cfblk7/1 -> cfblk5/1
  cfblk1/1 -> cfblk12/2(cfblk11)
  cfblk11/1(cfblk2) -> cfblk3/1
  cfblk9/2(cfblk17) -> cfblk4/1
  cfblk6/1 -> cfblk9/3(cfblk14), cfblk11/4(cfblk15)
  cfblk4/1 -> cfblk10/2(cfblk7)
  cfblk5/1 -> cfblk9/4(cfblk15)
  cfblk8/1 -> cfblk10/3(cfblk8)
  cfblk15/1 -> cfblk12/1(cfblk1)
  cfblk16/1 -> cfblk9/1(cfblk1)
  cfblk17/1 -> cfblk11/3(cfblk14)
  cfblk18/1 -> cfblk9/5(cfblk16)
  cfblk11/2(cfblk16) -> cfblk19/1
  cfblk19/1 -> cfblk10/1(cfblk1)

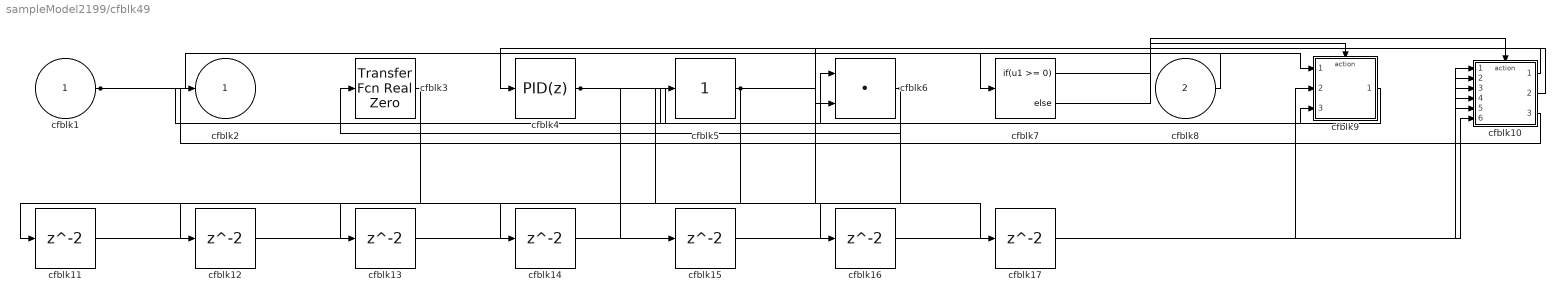
== system sampleModel2199/cfblk49 ==
  cfblk1 : Inport
  cfblk8 : Inport  Port=2
  cfblk10 : Subsystem  TreatAsAtomicUnit=on
  cfblk{11..17} (7 alike) : Delay  SampleTime=1
  cfblk3 : simulink/Discrete/Transfer Fcn Real Zero  ZeroZ=0.75  ICPrevInput=0.0  DoSatur=off
      settings: SourceProductBaseCode=SL
  cfblk4 : slpidlib/PID Controller  Controller=PID  Form=Parallel  TimeDomain=Discrete-time  UseExternalTs=off  SampleTime=1  IntegratorMethod=Forward Euler  FilterMethod=Forward Euler  ControllerParametersSource=internal  P=1  I=1  UseKiTs=off  D=0  N=100  UseFilter=on  TunerSelectOption=Transfer Function Based (PID Tuner App)  InitialConditionSource=internal  InitialConditionForIntegrator=0  InitialConditionForFilter=0  DifferentiatorICPrevScaledInput=0  ExternalReset=none  TrackingMode=off  Kt=1  LimitOutput=off  SatLimitsSource=internal  UpperSaturationLimit=inf  LowerSaturationLimit=-inf  LinearizeAsGain=off  AntiWindupMode=none  Kb=1  POutMin=[]  POutMax=[]  IOutMin=[]  IOutMax=[]  DOutMin=[]  DOutMax=[]  NOutMin=[]  NOutMax=[]  SumOutMin=[]  SumOutMax=[]  SaturationOutMin=[]  SaturationOutMax=[]  PParamMin=[]  PParamMax=[]  IParamMin=[]  IParamMax=[]  DParamMin=[]  DParamMax=[]  NParamMin=[]  NParamMax=[]  KbParamMin=[]  KbParamMax=[]  KtParamMin=[]  KtParamMax=[]  KbOutMin=[]  KbOutMax=[]  KtOutMin=[]  KtOutMax=[]  IntegratorOutMin=[]  IntegratorOutMax=[]  FilterOutMin=[]  FilterOutMax=[]  SumI1OutMin=[]  SumI1OutMax=[]  SumI2OutMin=[]  SumI2OutMax=[]  SumI3OutMin=[]  SumI3OutMax=[]  SumI4OutMin=[]  SumI4OutMax=[]  SumDOutMin=[]  SumDOutMax=[]  DifferentiatorOutMin=[]  DifferentiatorOutMax=[]  FilterDiffOutCoefMin=[]  FilterDiffOutCoefMax=[]  ReciprocalOutMin=[]  ReciprocalOutMax=[]  SumDenOutMin=[]  SumDenOutMax=[]  SumNumOutMin=[]  SumNumOutMax=[]  DivideOutMin=[]  DivideOutMax=[]  UdiffTsProdOutMin=[]  UdiffTsProdOutMax=[]  NTsProdOutMin=[]  NTsProdOutMax=[]  UintegralTsProdOutMin=[]  UintegralTsProdOutMax=[]  UngainTsProdOutMin=[]  UngainTsProdOutMax=[]  IntegratorContinuousStateAttributes=''  IntegratorStateMustResolveToSignalObject=off  IntegratorRTWStateStorageClass=Auto  FilterContinuousStateAttributes=''  FilterStateMustResolveToSignalObject=off  FilterRTWStateStorageClass=Auto  ParallelPVariant=InternalParameters  IdealPVariant=Disabled  IVariant=InternalParameters  DVariant=InternalParameters  IntegratorVariant=Discrete  SatVariant=Disabled  AWVariant=Passthrough  PCopyVariant=Disabled  TRVariant=Disabled  FdbkBlocksVariant=Forward  IdealPFdbkVariant=Disabled  SatFdbkVariant=Disabled  DerivativeFilterVariant=ForwardEulerFilter  NVariant=InternalParameters  NCopyVariant=Disabled  FilterICVariant=InternalICsFilter  IntegratorICVariant=InternalICs  ExternalResetVariant=Disabled  TRSumVariant=Passthrough  SumFdbkVariant=Disabled  SumVariant=Sum_PID  TsampFilterVariant=InternalTs  TsampNgainVariant=Passthrough  TsampIntegralVariant=Passthrough  ExternalSaturationOutDataTypeStr=Inherit: Same as second input  aMode=0
  cfblk5 : simulink/Math Operations/Slider Gain  gain=1  low=0  high=2
  cfblk6 : DotProduct  OutDataTypeStr=Inherit: Inherit via internal rule
  cfblk7 : If  IfExpression=u1 >= 0  SampleTime=1
  cfblk9 : Subsystem  TreatAsAtomicUnit=on
  cfblk2 : Outport
  wires:
  cfblk1/1 -> cfblk9/1(cfblk1), cfblk9/3(cfblk10)
  cfblk4/1 -> cfblk6/1, cfblk15/1, cfblk16/1
  cfblk6/1 -> cfblk3/1, cfblk14/1
  cfblk10/1(cfblk2) -> cfblk6/2
  cfblk9/1(cfblk2) -> cfblk5/1
  cfblk8/1 -> cfblk7/1
  cfblk10/2(cfblk15) -> cfblk4/1
  cfblk5/1 -> cfblk11/1, cfblk12/1, cfblk17/1
  cfblk10/3(cfblk16) -> cfblk2/1
  cfblk7/1 -> cfblk9/Action
  cfblk7/2 -> cfblk10/Action
  cfblk11/1 -> cfblk9/2(cfblk9)
  cfblk12/1 -> cfblk10/2(cfblk10)
  cfblk3/1 -> cfblk13/1
  cfblk13/1 -> cfblk10/1(cfblk1)
  cfblk14/1 -> cfblk10/6(cfblk14)
  cfblk15/1 -> cfblk10/4(cfblk12)
  cfblk16/1 -> cfblk10/5(cfblk13)
  cfblk17/1 -> cfblk10/3(cfblk11)

== system sampleModel2199/cfblk50 ==
  cfblk1 : Inport
  cfblk10 : Inport  Port=2
  cfblk11 : Delay  SampleTime=1
  cfblk3 : simulink/Discrete/Transfer Fcn Real Zero  ZeroZ=0.75  ICPrevInput=0.0  DoSatur=off
      settings: SourceProductBaseCode=SL
  cfblk4 : DiscreteStateSpace
  cfblk5 : simulink/Discrete/Transfer Fcn Lead or Lag  PoleZ=0.95  ZeroZ=0.75  ICPrevOutput=0.0  ICPrevInput=0.0  DoSatur=off
      settings: SourceProductBaseCode=SL
  cfblk6 : Rounding
  cfblk7 : Sqrt  Operator=rSqrt  AlgorithmType=Newton-Raphson
  cfblk8 : Subsystem
  cfblk9 : Subsystem
  cfblk2 : Outport
  wires:
  cfblk10/1 -> cfblk9/1(cfblk1)
  cfblk8/1(cfblk2) -> cfblk3/1
  cfblk4/1 -> cfblk6/1
  cfblk9/1(cfblk2) -> cfblk5/1
  cfblk8/2(cfblk15) -> cfblk2/1
  cfblk3/1 -> cfblk4/1
  cfblk1/1 -> cfblk7/1
  cfblk5/1 -> cfblk8/2(cfblk14)
  cfblk7/1 -> cfblk9/2(cfblk10)
  cfblk6/1 -> cfblk11/1
  cfblk11/1 -> cfblk8/1(cfblk1)

== system sampleModel2199/cfblk51 ==
  cfblk1 : Inport
  cfblk3 : Product  Inputs=**
  cfblk4 : Product  Inputs=**
  cfblk5 : Sqrt  Operator=rSqrt  AlgorithmType=Newton-Raphson
  cfblk6 : Trigonometry
  cfblk7 : Sum  Inputs=-+
  cfblk8 : Delay  SampleTime=1
  cfblk2 : Outport
  wires:
  cfblk6/1 -> cfblk4/1, cfblk3/2
  cfblk1/1 -> cfblk6/1
  cfblk5/1 -> cfblk2/1
  cfblk4/1 -> cfblk5/1
  cfblk3/1 -> cfblk4/2, cfblk7/1, cfblk7/2
  cfblk7/1 -> cfblk8/1
  cfblk8/1 -> cfblk3/1

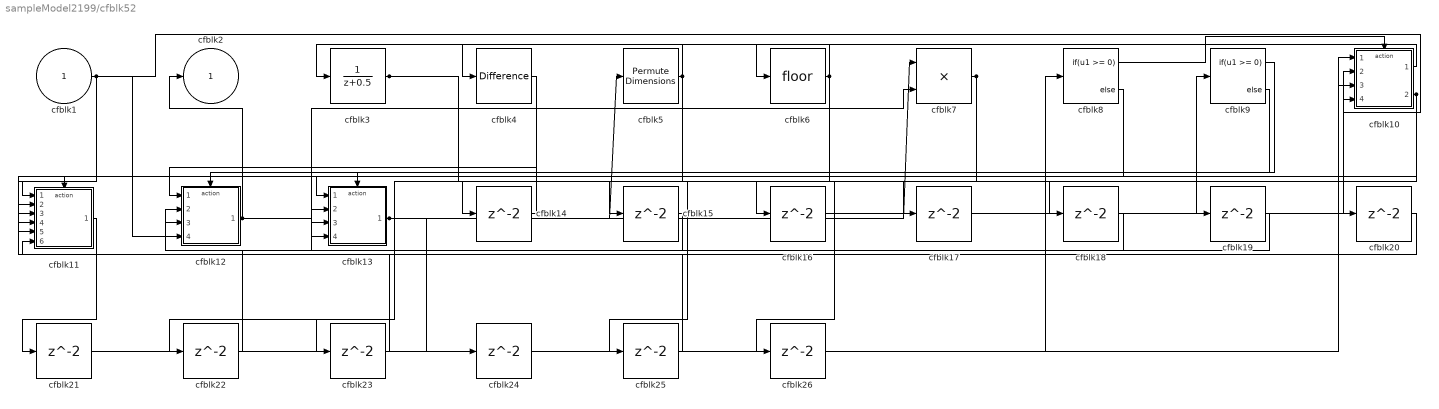
== system sampleModel2199/cfblk52 ==
  cfblk1 : Inport
  cfblk10 : Subsystem  TreatAsAtomicUnit=on
  cfblk11 : Subsystem  TreatAsAtomicUnit=on
  cfblk12 : Subsystem  TreatAsAtomicUnit=on
  cfblk13 : Subsystem  TreatAsAtomicUnit=on
  cfblk{14..26} (13 alike) : Delay  SampleTime=1
  cfblk3 : DiscreteTransferFcn  SampleTime=1
  cfblk4 : simulink/Discrete/Difference  ICPrevInput=0.0  OutMin=[]  OutMax=[]  OutDataTypeStr=Inherit: Inherit via back propagation  OutDataType=fixdt(1, 16)  OutScaling=2^-10  DoSatur=off
  cfblk5 : PermuteDimensions
  cfblk6 : Rounding
  cfblk7 : Product  Inputs=**
  cfblk8 : If  IfExpression=u1 >= 0  SampleTime=1
  cfblk9 : If  IfExpression=u1 >= 0  SampleTime=1
  cfblk2 : Outport
  wires:
  cfblk12/1(cfblk2) -> cfblk2/1, cfblk7/2
  cfblk4/1 -> cfblk13/1(cfblk1)
  cfblk3/1 -> cfblk17/1, cfblk18/1, cfblk19/1, cfblk20/1
  cfblk1/1 -> cfblk10/2(cfblk7), cfblk11/1(cfblk1), cfblk12/4(cfblk13), cfblk11/5(cfblk12)
  cfblk6/1 -> cfblk4/1, cfblk25/1
  cfblk13/1(cfblk2) -> cfblk5/1, cfblk7/1, cfblk24/1
  cfblk10/1(cfblk2) -> cfblk6/1
  cfblk7/1 -> cfblk14/1, cfblk15/1, cfblk16/1
  cfblk5/1 -> cfblk3/1, cfblk22/1, cfblk23/1
  cfblk10/2(cfblk10) -> cfblk11/2(cfblk9), cfblk13/4(cfblk12), cfblk26/1
  cfblk8/1 -> cfblk10/Action
  cfblk8/2 -> cfblk11/Action
  cfblk9/1 -> cfblk12/Action
  cfblk9/2 -> cfblk13/Action
  cfblk14/1 -> cfblk12/1(cfblk1)
  cfblk15/1 -> cfblk12/2(cfblk11)
  cfblk16/1 -> cfblk10/4(cfblk9)
  cfblk17/1 -> cfblk9/1
  cfblk18/1 -> cfblk13/2(cfblk10)
  cfblk19/1 -> cfblk13/3(cfblk11)
  cfblk20/1 -> cfblk11/4(cfblk11)
  cfblk11/1(cfblk2) -> cfblk21/1
  cfblk21/1 -> cfblk10/1(cfblk1)
  cfblk22/1 -> cfblk12/3(cfblk12)
  cfblk23/1 -> cfblk11/3(cfblk10)
  cfblk24/1 -> cfblk10/3(cfblk8)
  cfblk25/1 -> cfblk11/6(cfblk13)
  cfblk26/1 -> cfblk8/1

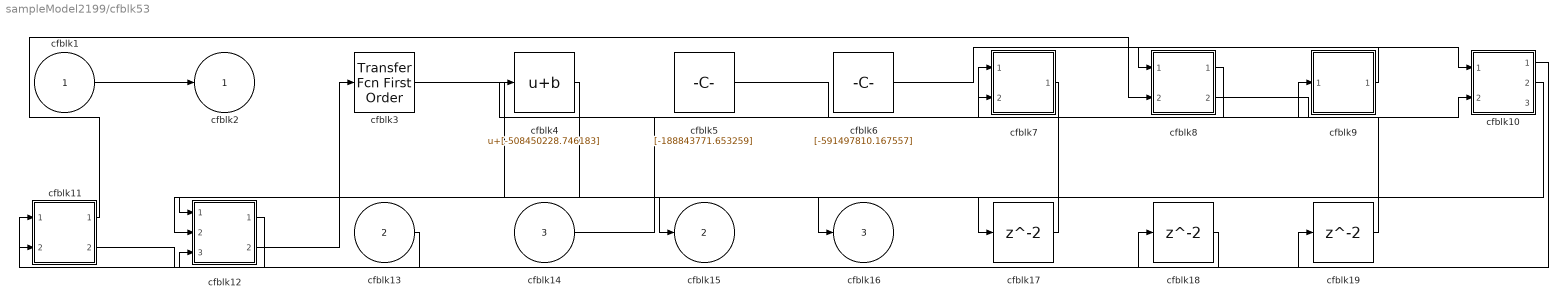
== system sampleModel2199/cfblk53 ==
  cfblk1 : Inport
  cfblk13 : Inport  Port=2
  cfblk14 : Inport  Port=3
  cfblk10 : Subsystem
  cfblk11 : Subsystem
  cfblk12 : Subsystem
  cfblk17 : Delay  SampleTime=1
  cfblk18 : Delay  SampleTime=1
  cfblk19 : Delay  SampleTime=1
  cfblk3 : simulink/Discrete/Transfer Fcn First Order  PoleZ=0.95  ICPrevOutput=0.0  DoSatur=off
  cfblk4 : Bias  Bias=[-508450228.746183]  SaturateOnIntegerOverflow=off
  cfblk5 : Constant  Value=[-188843771.653259]  SampleTime=1
  cfblk6 : Constant  Value=[-591497810.167557]  SampleTime=1
  cfblk7 : Subsystem
  cfblk8 : Subsystem
  cfblk9 : Subsystem
  cfblk2 : Outport
  cfblk15 : Outport  Port=2
  cfblk16 : Outport  Port=3
  wires:
  cfblk3/1 -> cfblk15/1
  cfblk5/1 -> cfblk7/1(cfblk1)
  cfblk12/1(cfblk2) -> cfblk11/1(cfblk1)
  cfblk13/1 -> cfblk11/2(cfblk8)
  cfblk12/2(cfblk9) -> cfblk3/1
  cfblk1/1 -> cfblk2/1
  cfblk9/1(cfblk2) -> cfblk8/1(cfblk1)
  cfblk11/1(cfblk2) -> cfblk8/2(cfblk11)
  cfblk6/1 -> cfblk10/1(cfblk1)
  cfblk8/1(cfblk2) -> cfblk7/2(cfblk7)
  cfblk8/2(cfblk12) -> cfblk10/2(cfblk13)
  cfblk4/1 -> cfblk12/2(cfblk7)
  cfblk10/2(cfblk14) -> cfblk16/1
  cfblk14/1 -> cfblk9/1(cfblk1)
  cfblk7/1(cfblk2) -> cfblk17/1
  cfblk17/1 -> cfblk12/1(cfblk1)
  cfblk10/1(cfblk2) -> cfblk18/1
  cfblk18/1 -> cfblk12/3(cfblk8)
  cfblk11/2(cfblk9) -> cfblk19/1
  cfblk19/1 -> cfblk4/1

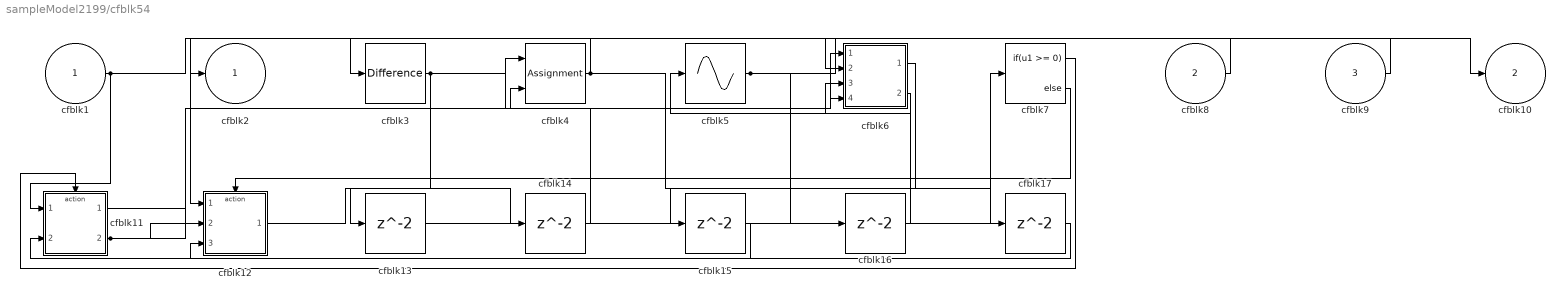
== system sampleModel2199/cfblk54 ==
  cfblk1 : Inport
  cfblk8 : Inport  Port=2
  cfblk9 : Inport  Port=3
  cfblk11 : Subsystem  TreatAsAtomicUnit=on
  cfblk12 : Subsystem  TreatAsAtomicUnit=on
  cfblk{13..17} (5 alike) : Delay  SampleTime=1
  cfblk3 : simulink/Discrete/Difference  ICPrevInput=0.0  OutMin=[]  OutMax=[]  OutDataTypeStr=Inherit: Inherit via back propagation  OutDataType=fixdt(1, 16)  OutScaling=2^-10  DoSatur=off
  cfblk4 : Assignment  DiagnosticForDimensions=Warning  IndexOptions=Index vector (dialog)  Indices=1  OutputSizes=1
  cfblk5 : Sin  TimeSource=Use external signal  SampleTime=0
  cfblk6 : Subsystem
  cfblk7 : If  IfExpression=u1 >= 0  SampleTime=1
  cfblk2 : Outport
  cfblk10 : Outport  Port=2
  wires:
  cfblk1/1 -> cfblk11/1(cfblk1), cfblk6/2(cfblk11)
  cfblk6/2(cfblk14) -> cfblk5/1
  cfblk8/1 -> cfblk12/1(cfblk1)
  cfblk3/1 -> cfblk6/4(cfblk13), cfblk13/1
  cfblk5/1 -> cfblk10/1, cfblk16/1
  cfblk9/1 -> cfblk2/1
  cfblk11/1(cfblk2) -> cfblk4/2
  cfblk4/1 -> cfblk3/1, cfblk17/1
  cfblk11/2(cfblk10) -> cfblk6/1(cfblk1), cfblk12/2(cfblk7)
  cfblk7/1 -> cfblk11/Action
  cfblk7/2 -> cfblk12/Action
  cfblk13/1 -> cfblk7/1
  cfblk12/1(cfblk2) -> cfblk14/1
  cfblk14/1 -> cfblk4/1
  cfblk6/1(cfblk2) -> cfblk15/1
  cfblk15/1 -> cfblk11/2(cfblk9)
  cfblk16/1 -> cfblk6/3(cfblk12)
  cfblk17/1 -> cfblk12/3(cfblk8)

== system sampleModel2199/cfblk55 ==
  cfblk1 : Inport
  cfblk{10..16} (7 alike) : Delay  SampleTime=1
  cfblk3 : simulink/Discrete/Transfer Fcn Real Zero  ZeroZ=0.75  ICPrevInput=0.0  DoSatur=off
      settings: SourceProductBaseCode=SL
  cfblk4 : simulink/Discrete/Tapped Delay  vinit=0.0  samptime=-1  NumDelays=1  DelayOrder=Oldest  includeCurrent=off
  cfblk5 : Subsystem
  cfblk6 : Subsystem
  cfblk7 : Subsystem
  cfblk8 : Subsystem
  cfblk9 : Subsystem
  cfblk2 : Outport
  wires:
  cfblk8/1(cfblk2) -> cfblk4/1
  cfblk9/1(cfblk2) -> cfblk8/1(cfblk1)
  cfblk1/1 -> cfblk2/1, cfblk6/1(cfblk1)
  cfblk3/1 -> cfblk7/2(cfblk10), cfblk11/1, cfblk12/1
  cfblk5/1(cfblk2) -> cfblk7/1(cfblk1), cfblk15/1, cfblk16/1
  cfblk4/1 -> cfblk3/1, cfblk10/1
  cfblk6/1(cfblk2) -> cfblk9/2(cfblk7), cfblk7/3(cfblk11)
  cfblk8/2(cfblk15) -> cfblk5/1(cfblk1)
  cfblk10/1 -> cfblk9/1(cfblk1)
  cfblk11/1 -> cfblk8/2(cfblk12)
  cfblk12/1 -> cfblk6/2(cfblk11)
  cfblk7/1(cfblk2) -> cfblk13/1
  cfblk13/1 -> cfblk8/3(cfblk13)
  cfblk7/2(cfblk12) -> cfblk14/1
  cfblk14/1 -> cfblk9/3(cfblk8)
  cfblk15/1 -> cfblk8/4(cfblk14)
  cfblk16/1 -> cfblk6/3(cfblk12)

== system sampleModel2199/cfblk56 ==
  cfblk1 : Inport
  cfblk10 : Delay  SampleTime=1
  cfblk3 : Math  Operator=log
  cfblk4 : UnaryMinus
  cfblk5 : ComplexToMagnitudeAngle
  cfblk6 : Constant  Value=[-529374541.402075]  SampleTime=1
  cfblk7 : Subsystem
  cfblk8 : Subsystem
  cfblk9 : Delay  SampleTime=1
  cfblk2 : Outport
  wires:
  cfblk3/1 -> cfblk2/1
  cfblk8/1(cfblk2) -> cfblk3/1
  cfblk7/1(cfblk2) -> cfblk5/1
  cfblk1/1 -> cfblk7/1(cfblk1)
  cfblk6/1 -> cfblk4/1
  cfblk7/2(cfblk14) -> cfblk8/1(cfblk1)
  cfblk4/1 -> cfblk7/4(cfblk13)
  cfblk5/1 -> cfblk9/1
  cfblk9/1 -> cfblk7/2(cfblk11)
  cfblk5/2 -> cfblk10/1
  cfblk10/1 -> cfblk7/3(cfblk12)

== system sampleModel2199/cfblk40/cfblk10 ==
  cfblk1 : Inport
  cfblk15 : Inport  Port=2
  cfblk10 : simulink/Math Operations/MinMax Running Resettable  Function=min  vinit=0.0
  cfblk11 : Polyval  Coefs=[ +2.081618890e-019, -1.441693666e-014, +4.719686976e-010, -8.536869453e-006, +1.621573104e-001, -8.087801117e+001 ]
  cfblk12 : Constant  Value=[952526584.303405]  SampleTime=1
  cfblk13 : Constant  Value=[-595387779.180219]  SampleTime=1
  cfblk14 : Constant  Value=[-781840086.265192]  SampleTime=1
  cfblk3 : Delay  ShowEnablePort=on  SampleTime=1
      settings: InputPortMap=u0,e6
  cfblk4 : UnitDelay  HasFrameUpgradeWarning=on
  cfblk5 : Gain  Gain=[413253760.549486]
  cfblk6 : Abs  SaturateOnIntegerOverflow=off
  cfblk7 : Sqrt  Operator=rSqrt  AlgorithmType=Newton-Raphson
  cfblk8 : simulink/Math Operations/Slider Gain  gain=1  low=0  high=2
  cfblk9 : Sum  Inputs=+
  cfblk2 : Outport
  wires:
  cfblk5/1 -> cfblk10/1
  cfblk14/1 -> cfblk4/1
  cfblk15/1 -> cfblk11/1
  cfblk3/1 -> cfblk6/1
  cfblk4/1 -> cfblk8/1
  cfblk1/1 -> cfblk10/2
  cfblk6/1 -> cfblk9/1
  cfblk10/1 -> cfblk3/1
  cfblk7/1 -> cfblk3/2
  cfblk11/1 -> cfblk5/1
  cfblk12/1 -> cfblk7/1
  cfblk9/1 -> cfblk2/1

== system sampleModel2199/cfblk40/cfblk11 ==
  cfblk1 : Inport
  cfblk9 : Inport  Port=2
  cfblk10 : Inport  Port=3
  cfblk11 : Inport  Port=4
  cfblk12 : Inport  Port=5
  cfblk13 : Delay  SampleTime=1
  cfblk3 : simulink/Discrete/Difference  ICPrevInput=0.0  OutMin=[]  OutMax=[]  OutDataTypeStr=Inherit: Inherit via back propagation  OutDataType=fixdt(1, 16)  OutScaling=2^-10  DoSatur=off
  cfblk4 : Polyval  Coefs=[ +2.081618890e-019, -1.441693666e-014, +4.719686976e-010, -8.536869453e-006, +1.621573104e-001, -8.087801117e+001 ]
  cfblk5 : MinMax  Function=max
  cfblk6 : Squeeze
  cfblk7 : Sqrt
  cfblk8 : Constant  Value=[-591060991.344899]  SampleTime=1
  cfblk2 : Outport
  wires:
  cfblk1/1 -> cfblk2/1
  cfblk9/1 -> cfblk7/1
  cfblk3/1 -> cfblk5/1
  cfblk5/1 -> cfblk6/1
  cfblk12/1 -> cfblk4/1
  cfblk6/1 -> cfblk13/1
  cfblk13/1 -> cfblk3/1

== system sampleModel2199/cfblk40/cfblk12 ==
  cfblk1 : Inport
  cfblk11 : Inport  Port=2
  cfblk10 : Constant  Value=[-565754399.400377]  SampleTime=1
  cfblk12 : Delay  SampleTime=1
  cfblk13 : Delay  SampleTime=1
  cfblk3 : slpidlib/PID Controller  Controller=PID  Form=Parallel  TimeDomain=Discrete-time  UseExternalTs=off  SampleTime=1  IntegratorMethod=Forward Euler  FilterMethod=Forward Euler  ControllerParametersSource=internal  P=1  I=1  UseKiTs=off  D=0  N=100  UseFilter=on  TunerSelectOption=Transfer Function Based (PID Tuner App)  InitialConditionSource=internal  InitialConditionForIntegrator=0  InitialConditionForFilter=0  DifferentiatorICPrevScaledInput=0  ExternalReset=none  TrackingMode=off  Kt=1  LimitOutput=off  SatLimitsSource=internal  UpperSaturationLimit=inf  LowerSaturationLimit=-inf  LinearizeAsGain=off  AntiWindupMode=none  Kb=1  POutMin=[]  POutMax=[]  IOutMin=[]  IOutMax=[]  DOutMin=[]  DOutMax=[]  NOutMin=[]  NOutMax=[]  SumOutMin=[]  SumOutMax=[]  SaturationOutMin=[]  SaturationOutMax=[]  PParamMin=[]  PParamMax=[]  IParamMin=[]  IParamMax=[]  DParamMin=[]  DParamMax=[]  NParamMin=[]  NParamMax=[]  KbParamMin=[]  KbParamMax=[]  KtParamMin=[]  KtParamMax=[]  KbOutMin=[]  KbOutMax=[]  KtOutMin=[]  KtOutMax=[]  IntegratorOutMin=[]  IntegratorOutMax=[]  FilterOutMin=[]  FilterOutMax=[]  SumI1OutMin=[]  SumI1OutMax=[]  SumI2OutMin=[]  SumI2OutMax=[]  SumI3OutMin=[]  SumI3OutMax=[]  SumI4OutMin=[]  SumI4OutMax=[]  SumDOutMin=[]  SumDOutMax=[]  DifferentiatorOutMin=[]  DifferentiatorOutMax=[]  FilterDiffOutCoefMin=[]  FilterDiffOutCoefMax=[]  ReciprocalOutMin=[]  ReciprocalOutMax=[]  SumDenOutMin=[]  SumDenOutMax=[]  SumNumOutMin=[]  SumNumOutMax=[]  DivideOutMin=[]  DivideOutMax=[]  UdiffTsProdOutMin=[]  UdiffTsProdOutMax=[]  NTsProdOutMin=[]  NTsProdOutMax=[]  UintegralTsProdOutMin=[]  UintegralTsProdOutMax=[]  UngainTsProdOutMin=[]  UngainTsProdOutMax=[]  IntegratorContinuousStateAttributes=''  IntegratorStateMustResolveToSignalObject=off  IntegratorRTWStateStorageClass=Auto  FilterContinuousStateAttributes=''  FilterStateMustResolveToSignalObject=off  FilterRTWStateStorageClass=Auto  ParallelPVariant=InternalParameters  IdealPVariant=Disabled  IVariant=InternalParameters  DVariant=InternalParameters  IntegratorVariant=Discrete  SatVariant=Disabled  AWVariant=Passthrough  PCopyVariant=Disabled  TRVariant=Disabled  FdbkBlocksVariant=Forward  IdealPFdbkVariant=Disabled  SatFdbkVariant=Disabled  DerivativeFilterVariant=ForwardEulerFilter  NVariant=InternalParameters  NCopyVariant=Disabled  FilterICVariant=InternalICsFilter  IntegratorICVariant=InternalICs  ExternalResetVariant=Disabled  TRSumVariant=Passthrough  SumFdbkVariant=Disabled  SumVariant=Sum_PID  TsampFilterVariant=InternalTs  TsampNgainVariant=Passthrough  TsampIntegralVariant=Passthrough  ExternalSaturationOutDataTypeStr=Inherit: Same as second input  aMode=0
  cfblk4 : Squeeze
  cfblk5 : Sum  Inputs=+-
  cfblk6 : MinMax  Inputs=3
  cfblk7 : Sum
  cfblk8 : ComplexToMagnitudeAngle
  cfblk9 : Sum  Inputs=+-
  cfblk2 : Outport
  wires:
  cfblk5/1 -> cfblk6/1, cfblk3/1
  cfblk7/1 -> cfblk8/1
  cfblk1/1 -> cfblk4/1
  cfblk3/1 -> cfblk2/1, cfblk6/3
  cfblk4/1 -> cfblk5/1
  cfblk10/1 -> cfblk7/2
  cfblk8/2 -> cfblk9/1
  cfblk6/1 -> cfblk9/2
  cfblk11/1 -> cfblk5/2
  cfblk9/1 -> cfblk12/1
  cfblk12/1 -> cfblk6/2
  cfblk8/1 -> cfblk13/1
  cfblk13/1 -> cfblk7/1

== system sampleModel2199/cfblk40/cfblk13 ==
  cfblk1 : Inport
  cfblk11 : Inport  Port=2
  cfblk12 : Inport  Port=3
  cfblk10 : Constant  Value=[-534732202.956618]  SampleTime=1
  cfblk3 : simulink/Discrete/Difference  ICPrevInput=0.0  OutMin=[]  OutMax=[]  OutDataTypeStr=Inherit: Inherit via back propagation  OutDataType=fixdt(1, 16)  OutScaling=2^-10  DoSatur=off
  cfblk4 : simulink/Discrete/Transfer Fcn Lead or Lag  PoleZ=0.95  ZeroZ=0.75  ICPrevOutput=0.0  ICPrevInput=0.0  DoSatur=off
      settings: SourceProductBaseCode=SL
  cfblk5 : DiscreteIntegrator  ICPrevOutput=DiscIntNeverNeededParam  ICPrevScaledInput=DiscIntNeverNeededParam
  cfblk6 : MinMax  Inputs=2
  cfblk7 : Sqrt  Operator=rSqrt  AlgorithmType=Newton-Raphson
  cfblk8 : ComplexToMagnitudeAngle
  cfblk9 : Constant  Value=[-147095149.173139]  SampleTime=1
  cfblk2 : Outport
  wires:
  cfblk7/1 -> cfblk3/1
  cfblk11/1 -> cfblk7/1
  cfblk10/1 -> cfblk4/1
  cfblk12/1 -> cfblk2/1
  cfblk5/1 -> cfblk8/1
  cfblk9/1 -> cfblk6/1
  cfblk3/1 -> cfblk5/1
  cfblk4/1 -> cfblk6/2

== system sampleModel2199/cfblk41/cfblk10 ==
  cfblk1 : Inport
  cfblk11 : Inport  Port=2
  cfblk12 : Inport  Port=3
  cfblk10 : Constant  Value=[-830285415.243033]  SampleTime=1
  cfblk3 : DiscreteZeroPole  Poles=[0 0.5]  Gain=1
  cfblk4 : DiscreteZeroPole  Poles=[0 0.5]  Gain=1
  cfblk5 : simulink/Discrete/Transfer Fcn Lead or Lag  PoleZ=0.95  ZeroZ=0.75  ICPrevOutput=0.0  ICPrevInput=0.0  DoSatur=off
      settings: SourceProductBaseCode=SL
  cfblk6 : ComplexToMagnitudeAngle
  cfblk7 : DotProduct  OutDataTypeStr=Inherit: Inherit via internal rule
  cfblk8 : Sum  Inputs=+-
  cfblk9 : Constant  Value=[985327650.465732]  SampleTime=1
  cfblk2 : Outport
  cfblk13 : Outport  Port=2
  cfblk14 : Outport  Port=3
  wires:
  cfblk10/1 -> cfblk8/1
  cfblk3/1 -> cfblk7/1
  cfblk11/1 -> cfblk3/1
  cfblk12/1 -> cfblk7/2
  cfblk1/1 -> cfblk13/1
  cfblk7/1 -> cfblk14/1
  cfblk6/1 -> cfblk4/1
  cfblk9/1 -> cfblk8/2
  cfblk5/1 -> cfblk2/1
  cfblk8/1 -> cfblk6/1
  cfblk4/1 -> cfblk5/1

== system sampleModel2199/cfblk41/cfblk11 ==
  cfblk1 : Inport
  cfblk12 : Inport  Port=2
  cfblk13 : Inport  Port=3
  cfblk14 : Inport  Port=4
  cfblk10 : Product
  cfblk11 : Constant  Value=[-401512766.162783]  SampleTime=1
  cfblk3 : UnitDelay  HasFrameUpgradeWarning=on
  cfblk4 : simulink/Discrete/Transfer Fcn Real Zero  ZeroZ=0.75  ICPrevInput=0.0  DoSatur=off
      settings: SourceProductBaseCode=SL
  cfblk5 : simulink/Discrete/Transfer Fcn Real Zero  ZeroZ=0.75  ICPrevInput=0.0  DoSatur=off
      settings: SourceProductBaseCode=SL
  cfblk6 : Reshape
  cfblk7 : Product  Inputs=*
  cfblk8 : Rounding
  cfblk9 : ComplexToRealImag
  cfblk2 : Outport
  cfblk15 : Outport  Port=2
  wires:
  cfblk6/1 -> cfblk4/1
  cfblk10/1 -> cfblk15/1
  cfblk14/1 -> cfblk6/1
  cfblk11/1 -> cfblk5/1
  cfblk5/1 -> cfblk10/1
  cfblk4/1 -> cfblk10/2
  cfblk9/1 -> cfblk8/1
  cfblk13/1 -> cfblk3/1
  cfblk9/2 -> cfblk7/1
  cfblk12/1 -> cfblk9/1
  cfblk3/1 -> cfblk2/1

== system sampleModel2199/cfblk41/cfblk12 ==
  cfblk1 : Inport
  cfblk11 : Inport  Port=2
  cfblk12 : Inport  Port=3
  cfblk10 : Constant  Value=[802351818.074435]  SampleTime=1
  cfblk3 : simulink/Discrete/Transfer Fcn First Order  PoleZ=0.95  ICPrevOutput=0.0  DoSatur=off
  cfblk4 : DiscreteStateSpace
  cfblk5 : UnaryMinus
  cfblk6 : Sqrt  Operator=rSqrt  AlgorithmType=Newton-Raphson
  cfblk7 : ComplexToRealImag
  cfblk8 : simulink/Math Operations/MinMax Running Resettable  Function=min  vinit=0.0
  cfblk9 : Constant  Value=[663552764.814756]  SampleTime=1
  cfblk2 : Outport
  wires:
  cfblk1/1 -> cfblk7/1
  cfblk10/1 -> cfblk6/1
  cfblk7/1 -> cfblk4/1
  cfblk9/1 -> cfblk2/1
  cfblk6/1 -> cfblk3/1
  cfblk3/1 -> cfblk8/1
  cfblk7/2 -> cfblk5/1
  cfblk11/1 -> cfblk8/2

== system sampleModel2199/cfblk43/cfblk7 ==
  cfblk1 : Inport
  cfblk8 : Inport  Port=2
  cfblk9 : Inport  Port=3
  cfblk10 : Inport  Port=4
  cfblk11 : Inport  Port=5
  cfblk3 : Trigonometry
  cfblk4 : MinMax  Function=max
  cfblk5 : UnaryMinus
  cfblk6 : PermuteDimensions
  cfblk7 : Constant  Value=[618720681.914850]  SampleTime=1
  cfblk2 : Outport
  cfblk12 : Outport  Port=2
  cfblk13 : Outport  Port=3
  cfblk14 : Outport  Port=4
  wires:
  cfblk11/1 -> cfblk12/1
  cfblk5/1 -> cfblk14/1
  cfblk1/1 -> cfblk6/1
  cfblk7/1 -> cfblk3/1
  cfblk8/1 -> cfblk2/1
  cfblk9/1 -> cfblk4/1
  cfblk3/1 -> cfblk13/1
  cfblk4/1 -> cfblk5/1

== system sampleModel2199/cfblk44/cfblk5 ==
  cfblk1 : Inport
  cfblk7 : Inport  Port=2
  cfblk8 : Inport  Port=3
  cfblk11 : Delay  SampleTime=1
  cfblk3 : simulink/Discrete/Difference  ICPrevInput=0.0  OutMin=[]  OutMax=[]  OutDataTypeStr=Inherit: Inherit via back propagation  OutDataType=fixdt(1, 16)  OutScaling=2^-10  DoSatur=off
  cfblk4 : PermuteDimensions
  cfblk5 : DotProduct  OutDataTypeStr=Inherit: Inherit via internal rule
  cfblk6 : Sum  Inputs=+-
  cfblk2 : Outport
  cfblk9 : Outport  Port=2
  cfblk10 : Outport  Port=3
  wires:
  cfblk8/1 -> cfblk3/1
  cfblk1/1 -> cfblk10/1
  cfblk3/1 -> cfblk2/1
  cfblk4/1 -> cfblk5/1, cfblk6/2
  cfblk7/1 -> cfblk6/1
  cfblk6/1 -> cfblk5/2, cfblk9/1
  cfblk5/1 -> cfblk11/1
  cfblk11/1 -> cfblk4/1

== system sampleModel2199/cfblk44/cfblk6 ==
  cfblk1 : Inport
  cfblk13 : Inport  Port=2
  cfblk14 : Inport  Port=3
  cfblk15 : Inport  Port=4
  cfblk16 : Inport  Port=5
  cfblk10 : Product  Inputs=*
  cfblk11 : Product  Inputs=**
  cfblk12 : Assignment  DiagnosticForDimensions=Warning  IndexOptions=Index vector (dialog)  Indices=1  OutputSizes=1
  cfblk3 : DiscreteIntegrator  ICPrevOutput=DiscIntNeverNeededParam  ICPrevScaledInput=DiscIntNeverNeededParam
  cfblk4 : simulink/Discrete/Difference  ICPrevInput=0.0  OutMin=[]  OutMax=[]  OutDataTypeStr=Inherit: Inherit via back propagation  OutDataType=fixdt(1, 16)  OutScaling=2^-10  DoSatur=off
  cfblk5 : simulink/Discrete/Difference  ICPrevInput=0.0  OutMin=[]  OutMax=[]  OutDataTypeStr=Inherit: Inherit via back propagation  OutDataType=fixdt(1, 16)  OutScaling=2^-10  DoSatur=off
  cfblk6 : UnitDelay  HasFrameUpgradeWarning=on
  cfblk7 : simulink/Math Operations/Slider Gain  gain=1  low=0  high=2
  cfblk8 : Abs  SaturateOnIntegerOverflow=off
  cfblk9 : Sin  TimeSource=Use external signal  SampleTime=0
  cfblk2 : Outport
  cfblk17 : Outport  Port=2
  wires:
  cfblk13/1 -> cfblk6/1
  cfblk14/1 -> cfblk12/1
  cfblk1/1 -> cfblk2/1
  cfblk8/1 -> cfblk9/1
  cfblk3/1 -> cfblk4/1
  cfblk5/1 -> cfblk3/1
  cfblk10/1 -> cfblk11/1
  cfblk4/1 -> cfblk12/2
  cfblk9/1 -> cfblk5/1
  cfblk11/1 -> cfblk8/1
  cfblk15/1 -> cfblk17/1
  cfblk6/1 -> cfblk7/1
  cfblk7/1 -> cfblk11/2
  cfblk16/1 -> cfblk10/1

== system sampleModel2199/cfblk45/cfblk12 ==
  cfblk1 : Inport
  cfblk9 : Inport  Port=2
  cfblk10 : Inport  Port=3
  cfblk11 : Inport  Port=4
  cfblk12 : Inport  Port=5
  cfblk3 : UnitDelay  HasFrameUpgradeWarning=on
  cfblk4 : DiscreteIntegrator  ICPrevOutput=DiscIntNeverNeededParam  ICPrevScaledInput=DiscIntNeverNeededParam
  cfblk5 : DiscreteStateSpace
  cfblk6 : Math
  cfblk7 : ComplexToRealImag
  cfblk8 : Squeeze
  cfblk2 : Outport
  cfblk13 : Outport  Port=2
  cfblk14 : Outport  Port=3
  wires:
  cfblk10/1 -> cfblk8/1
  cfblk9/1 -> cfblk3/1
  cfblk12/1 -> cfblk5/1
  cfblk8/1 -> cfblk4/1
  cfblk5/1 -> cfblk6/1
  cfblk7/1 -> cfblk14/1
  cfblk3/1 -> cfblk2/1
  cfblk4/1 -> cfblk7/1
  cfblk11/1 -> cfblk13/1

== system sampleModel2199/cfblk45/cfblk13 ==
  cfblk1 : Inport
  cfblk10 : Inport  Port=2
  cfblk11 : Inport  Port=3
  cfblk12 : Delay  SampleTime=1
  cfblk3 : Sqrt
  cfblk4 : Sqrt
  cfblk5 : Product  Inputs=*
  cfblk6 : Sum  Inputs=|++
  cfblk7 : PermuteDimensions
  cfblk8 : Constant  Value=[-525723442.783271]  SampleTime=1
  cfblk9 : Constant  Value=[972453737.987159]  SampleTime=1
  cfblk2 : Outport
  wires:
  cfblk5/1 -> cfblk6/1
  cfblk11/1 -> cfblk4/1
  cfblk9/1 -> cfblk7/1
  cfblk10/1 -> cfblk3/1
  cfblk8/1 -> cfblk6/2
  cfblk3/1 -> cfblk2/1
  cfblk6/1 -> cfblk12/1
  cfblk12/1 -> cfblk5/1
